simulink model "ControleEE_ObsPert"  (R2022b)
settings: Solver=ode45  StartTime=0.0  StopTime=30  RelTol=1e-6  EnableMultiTasking=on
values from neighbouring files (symbols this model uses):
  K = acker(A,B,p)    [PrObsPertContinuoRed.m]    (also in PrPara2nl_PI.m = acker(Aa,Ba,[p,p,p]); TestesEE.m = acker(A,B,[p,p,p]); TestesEEcanalI.m = acker(A,B,[p,-.6-1.0198i,-.6+1.0198i]); TestesEEobsPert.m = acker(A,B,[p,-.6-1.0198i,-.6+1.0198i]))
  L = L'    [PrObsPertContinuoRed.m]    (also in PrPara2nl_PI.m; TestesEE.m; TestesEEcanalI.m; TestesEEobsPert.m)
  Nb = gf.den{1}(1,2)/gf.num{1}(1,2)    [PrObsPertContinuoRed.m]    (also in PrPara2nl_PI.m = gf.den{1}(1,3)/gf.num{1}(1,3); TestesEE.m = gf.den{1}(1,4)/gf.num{1}(1,4); TestesEEcanalI.m = gf.den{1}(1,4)/gf.num{1}(1,4); TestesEEobsPert.m = gf.den{1}(1,4)/gf.num{1}(1,4))
  w0 = .5    (= 0.5)    [PrObsPertContinuoRed.m]    (also in TestesEEobsPert.m)
settings Model: Creator=Adolfo  LastModifiedBy=adolfo
settings SolverCC: AlgebraicLoopSolver=TrustRegion
settings DataIOCC: LimitDataPoints=on  SaveFormat=Array  SignalLoggingSaveFormat=ModelDataLogs  ReturnWorkspaceOutputs=off
settings OptimizationCC: ExpressionDepthLimit=2147483647  InitFltsAndDblsToZero=on  LifeSpan=inf
settings DebuggingCC: SaveWithParameterizedLinksMsg=none  UnderspecifiedInitializationDetection=Classic  MergeDetectMultiDrivingBlocksExec=none  SignalResolutionControl=TryResolveAllWithWarning  SolverPrmCheckMsg=warning  MultiTaskDSMMsg=warning  MultiTaskCondExecSysMsg=none  FcnCallInpInsideContextMsg=warning  UnconnectedInputMsg=warning  UnconnectedOutputMsg=warning  UnconnectedLineMsg=warning  StateNameClashWarn=warning  SFUnexpectedBacktrackingDiag=warning  SFNoUnconditionalDefaultTransitionDiag=warning  SFExecutionAtInitializationDiag=none  SFMachineParentedDataDiag=warning  ArithmeticOperatorsInVariantConditions=warning
settings HardwareCC: ProdBitPerPointer=32  ProdBitPerSizeT=32  ProdBitPerPtrDiffT=32  ProdLargestAtomicFloat=None  ProdIntDivRoundTo=Undefined  ProdEndianess=Unspecified  ProdWordSize=32  ProdHWDeviceType=32-bit Generic
settings ModelReferenceCC: EnableRefExpFcnMdlSchedulingChecks=on  PropagateSignalLabelsOutOfModel=off
settings SFSimCC: SimUseLocalCustomCode=off  CustomCodeUndefinedFunction=UseInterfaceOnly
settings RTWCC: RTWUseLocalCustomCode=off
settings CodeAppCC: StateflowObjectComments=on
settings GRTTargetCC: TargetFcnLib=ansi_tfl_tmw.mat  TargetLangStandard=C89/C90 (ANSI)  CombineOutputUpdateFcns=off  GRTInterface=on
settings ConfigComp: CovMetricSettings=dw  CovSaveCumulativeToWorkspaceVar=on  CovSaveSingleToWorkspaceVar=on  CovExternalEMLEnable=off  CovSFcnEnable=off

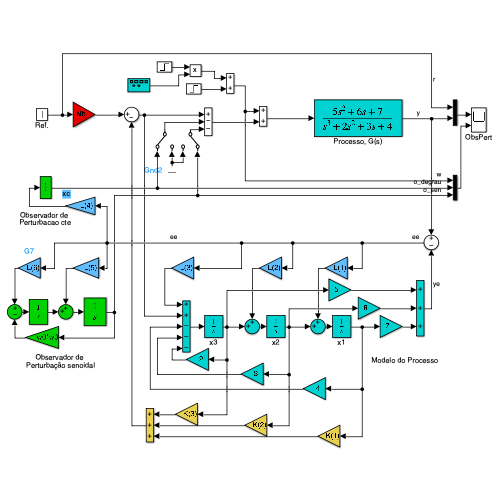
[thumbnail: Simulink's stored preview of the top-level diagram]
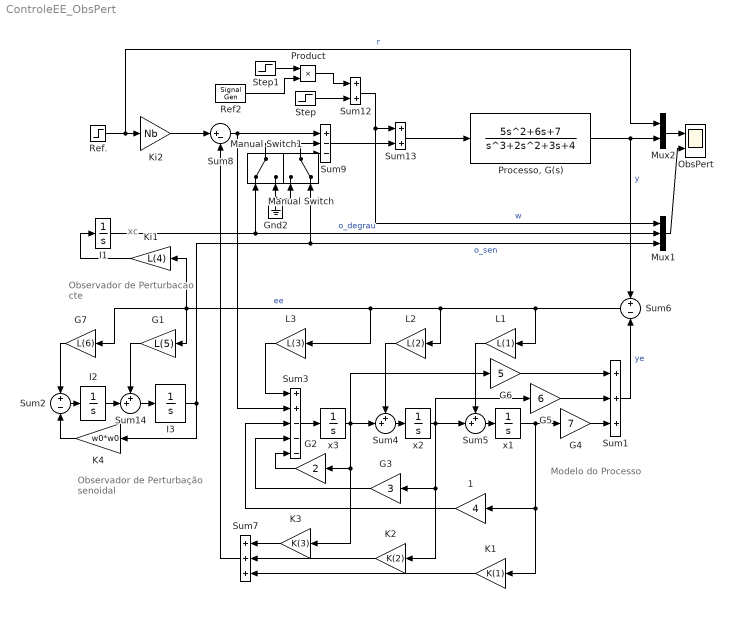
== system ControleEE_ObsPert ==
  note: xc
  note: Observador de
      | Perturbacao cte
  note: Observador de
      | Perturbação senoidal
  note: Modelo do Processo
  1 : Gain  Gain=4
  G1 : Gain  Gain=L(5)  SaturateOnIntegerOverflow=on  OutDataTypeStr=Inherit: Same as input  ParamDataTypeStr=Inherit: Same as input
  G2 : Gain  Gain=2
  G3 : Gain  Gain=3
  G4 : Gain  Gain=7
  G5 : Gain  Gain=6
  G6 : Gain  Gain=5
  G7 : Gain  Gain=L(6)  SaturateOnIntegerOverflow=on  OutDataTypeStr=Inherit: Same as input  ParamDataTypeStr=Inherit: Same as input
  Gnd2 : Ground
  I1 : Integrator
  I2 : Integrator
  I3 : Integrator
  K1 : Gain  Gain=K(1)
  K2 : Gain  Gain=K(2)
  K3 : Gain  Gain=K(3)
  K4 : Gain  Gain=w0*w0  SaturateOnIntegerOverflow=on  OutDataTypeStr=Inherit: Same as input  ParamDataTypeStr=Inherit: Same as input
  Ki1 : Gain  Gain=L(4)
  Ki2 : Gain  Gain=Nb
  L1 : Gain  Gain=L(1)
  L2 : Gain  Gain=L(2)
  L3 : Gain  Gain=L(3)
  Manual Switch : ManualSwitch  CurrentSetting=0
  Manual Switch1 : ManualSwitch
  Mux1 : Mux  Inputs=3
  Mux2 : Mux  Inputs=2
  ObsPert : Scope  NumInputPorts=2
  "Processo, G(s)" : TransferFcn  Numerator=[5 6 7]  Denominator=[1 2 3 4]
  Product : Product
  Ref. : Step  Time=0  SampleTime=0
  Ref2 : SignalGenerator  Amplitude=20  Frequency=w0  Units=rad/sec
  Step : Step  Time=3  After=3  SampleTime=0
  Step1 : Step  Time=2*pi/w0  SampleTime=0
  Sum1 : Sum  Inputs=+++
  Sum12 : Sum
  Sum13 : Sum
  Sum14 : Sum  Inputs=++|  InputSameDT=on  SaturateOnIntegerOverflow=on  OutDataTypeStr=Inherit: Same as first input
  Sum2 : Sum  Inputs=+-  InputSameDT=on  SaturateOnIntegerOverflow=on  OutDataTypeStr=Inherit: Same as first input
  Sum3 : Sum  Inputs=++---
  Sum4 : Sum  Inputs=++|
  Sum5 : Sum  Inputs=++|
  Sum6 : Sum  Inputs=+-
  Sum7 : Sum  Inputs=+++
  Sum8 : Sum  Inputs=|+-
  Sum9 : Sum  Inputs=+--
  x1 : Integrator
  x2 : Integrator
  x3 : Integrator
  wires:
  Ref./1 -> Mux2/1, Ki2/1  "r"
  Mux2/1 -> ObsPert/1
  x3/1 -> G6/1, Sum4/2, G2/1, K3/1
  x2/1 -> G5/1, Sum5/2, G3/1, K2/1
  Sum3/1 -> x3/1
  G2/1 -> Sum3/5
  G3/1 -> Sum3/4
  x1/1 -> G4/1, 1/1, K1/1
  1/1 -> Sum3/3
  G4/1 -> Sum1/3
  G5/1 -> Sum1/2
  G6/1 -> Sum1/1
  "Processo, G(s)"/1 -> Mux2/2, Sum6/1  "y"
  Sum1/1 -> Sum6/2  "ye"
  Sum13/1 -> "Processo, G(s)"/1
  Sum4/1 -> x2/1
  Sum5/1 -> x1/1
  L3/1 -> Sum3/1
  L2/1 -> Sum4/1
  L1/1 -> Sum5/1
  K3/1 -> Sum7/1
  K2/1 -> Sum7/2
  K1/1 -> Sum7/3
  Sum8/1 -> Sum3/2, Sum9/1
  Ki2/1 -> Sum8/1
  Sum7/1 -> Sum8/2
  Gnd2/1 -> Manual Switch/1, Manual Switch1/2
  Sum9/1 -> Sum13/2
  Manual Switch/1 -> Sum9/3
  Mux1/1 -> ObsPert/2
  Step/1 -> Sum12/2
  Sum12/1 -> Sum13/1, Mux1/1  "w"
  Manual Switch1/1 -> Sum9/2
  I1/1 -> Mux1/2, Manual Switch1/1  "o_degrau"
  Step1/1 -> Product/1
  Ref2/1 -> Product/2
  Ki1/1 -> I1/1
  Product/1 -> Sum12/1
  G1/1 -> Sum14/1
  I3/1 -> K4/1, Manual Switch/2, Mux1/3  "o_sen"
  G7/1 -> Sum2/1
  I2/1 -> Sum14/2
  Sum6/1 -> L2/1, Ki1/1, G7/1, G1/1, L3/1, L1/1  "ee"
  Sum14/1 -> I3/1
  Sum2/1 -> I2/1
  K4/1 -> Sum2/2
